simulink model "lab_2_4"  (R2024a)
settings: Solver=VariableStepAuto  StartTime=0.0  StopTime=50  MaxStep=1/128  RelTol=1e-3
settings Model: Creator=lw53894  LastModifiedBy=lw53894

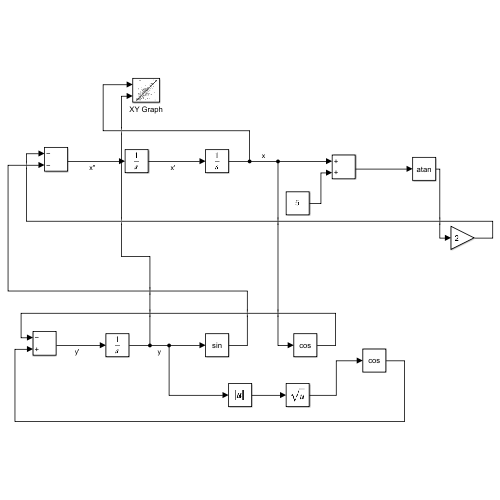
[thumbnail: Simulink's stored preview of the top-level diagram]
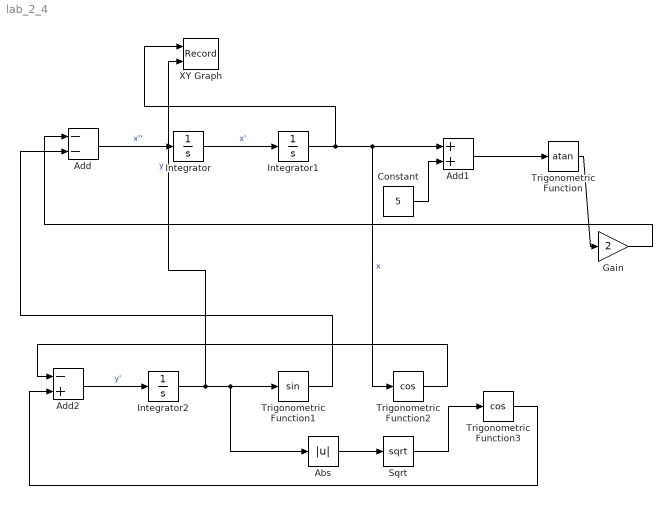
== system lab_2_4 ==
  Abs : Abs  SaturateOnIntegerOverflow=off
  Add : Sum  Inputs=--
  Add1 : Sum
  Add2 : Sum  Inputs=-+
  Constant : Constant  Value=5
  Gain : Gain  Gain=2
  Integrator : Integrator  InitialCondition=5
  Integrator1 : Integrator  InitialCondition=1
  Integrator2 : Integrator  InitialCondition=2
  Sqrt : Sqrt
  Trigonometric Function : Trigonometry  Operator=atan
  Trigonometric Function1 : Trigonometry
  Trigonometric Function2 : Trigonometry  Operator=cos
  Trigonometric Function3 : Trigonometry  Operator=cos
  XY Graph : Record  FileSettingsInternal="{\"entries\":[{\"content\":{\"excelSettings\":{\"content\":{},\"type\":\"Streamout.ExcelSettings\"}},\"type\":\"Streamout.FileSettingStorage\",\"uuid\":\"\"}],\"packageUris\":[\"http:\\/\\/schema.mathworks.com\\/mf0\\/streamout_blocks\\/R2020a\"],\"version\":\"1.0\"}"  Layout=[1 1]  SignalsInternal="{\"entries\":[{\"content\":{\"signals\":[{\"content\":{\"blockPath\":[],\"dimensions\":[1],\"domain\":\"\",\"lineColor\":\"#a2142f\",\"plots\":[ 1 ],\"port\":1,\"sid\":[\"\"],\"signalID\":1,\"signalName\":\"x\"},\"type\":\"RecordBlkView.Signal\",\"uuid\":\"\"},{\"content\":{\"blockPath\":[],\"dimensions\":[1],\"domain\":\"\",\"lineColor\":\"#139fff\",\"plots\":[ 1 ],\"port\":2,\"sid\":[\"\"],\"signalID\":2,\"signalName\":\"y\"},\"type\":\"RecordBlkView.Signal\",\"uuid\":\"\"}]},\"type\":\"RecordBlkView.InputSignals\",\"uuid\":\"\"}],\"packageUris\":[\"http:\\/\\/schema.mathworks.com\\/mf0\\/streamout_blocks\\/R2020a\"],\"version\":\"1.0\"}"  VisualizationBindings="{\"xyplotplugin\":{\"info\":[{\"series\":[{\"bindingParametersList\":[{\"parameter\":\"X-Axis\",\"signalID\":1,\"signalName\":\"x\"},{\"parameter\":\"Y-Axis\",\"signalID\":2,\"signalName\":\"y\"}],\"seriesID\":0}],\"subplotID\":1}]}}"  CompatibilityTag=XY
  wires:
  Integrator/1 -> Integrator1/1  "x'"
  Add/1 -> Integrator/1  "x''"
  Integrator1/1 -> XY Graph/1, Trigonometric Function2/1, Add1/1  "x"
  Constant/1 -> Add1/2
  Add1/1 -> Trigonometric Function/1
  Trigonometric Function/1 -> Gain/1
  Gain/1 -> Add/1
  Add2/1 -> Integrator2/1  "y'"
  Integrator2/1 -> XY Graph/2, Abs/1, Trigonometric Function1/1  "y"
  Trigonometric Function1/1 -> Add/2
  Trigonometric Function2/1 -> Add2/1
  Abs/1 -> Sqrt/1
  Sqrt/1 -> Trigonometric Function3/1
  Trigonometric Function3/1 -> Add2/2
